simulink model "TMR_Model"  (R2024a)
settings: Solver=FixedStepAuto  StartTime=0.0  StopTime=10.0  RelTol=1e-3
settings OptimizationCC: DefaultParameterBehavior=Inlined  UseDivisionForNetSlopeComputation=on  GainParamInheritBuiltInType=on  UseFloatMulNetSlope=on  InlineInvariantSignals=on  PassReuseOutputArgsAs=Individual arguments  ZeroExternalMemoryAtStartup=off  ZeroInternalMemoryAtStartup=off  NoFixptDivByZeroProtection=on  EfficientFloat2IntCast=on  LifeSpan=1  OptimizeBlockOrder=speed  DifferentSizesBufferReuse=on  EfficientTunableParamExpr=on
settings DebuggingCC: ParameterTunabilityLossMsg=error
settings HardwareCC: ProdBitPerInt=16  ProdBitPerPointer=16  ProdBitPerSizeT=16  ProdBitPerPtrDiffT=16  ProdLargestAtomicFloat=None  ProdWordSize=8  ProdLongLongMode=on  ProdHWDeviceType=Atmel->AVR
settings SFSimCC: MATLABDynamicMemAlloc=off
settings RTWCC: Description=Embedded Coder  SystemTargetFile=ert.tlc  TemplateMakefile=ert_default_tmf
settings CodeAppCC: ForceParamTrailComments=on  IgnoreCustomStorageClasses=off  OperatorAnnotations=on  SimulinkDataObjDesc=on  SFDataObjDesc=on  CustomSymbolStrGlobalVar=rt$N$M  CustomSymbolStrType=$N$M  CustomSymbolStrFcn=$N$M$F  CustomSymbolStrMacro=$N$M  InsertBlockDesc=on
settings ERTTargetCC: TargetLangStandard=C99 (ISO)  GenerateSampleERTMain=on  IncludeMdlTerminateFcn=off  CombineSignalStateStructs=on  SupportAbsoluteTime=off  SupportComplex=off  SupportContinuousTime=on  InlinedParameterPlacement=NonHierarchical  ERTCustomFileTemplate=example_file_process.tlc  ERTFilePackagingFormat=CompactWithDataFile

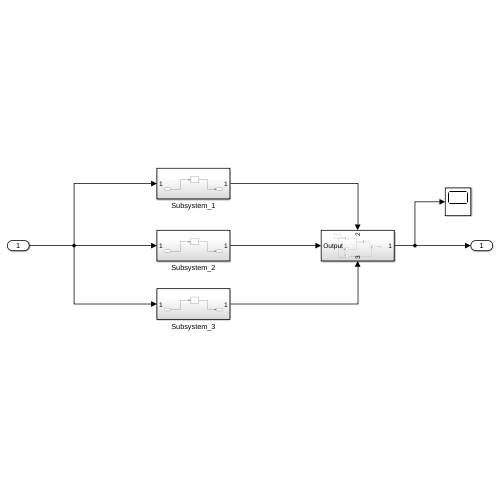
[thumbnail: Simulink's stored preview of the top-level diagram]
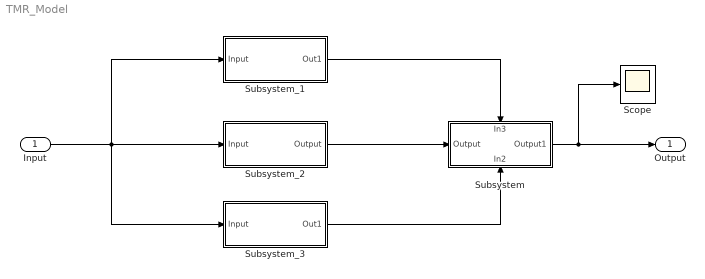
== system TMR_Model ==
  Input : Inport
  Scope : Scope
  Subsystem : Subsystem
      settings: PortSchema="{\"entries\":[{\"content\":{\"sides\":[{\"content\":{\"connectorIds\":[\"In1\"]},\"type\":\"ConnectorPlacement.EquallySpacedRectSide\",\"uuid\":\"1f9a2672-6573-4709-8234-f598f1a5eca2\"},{\"content\":{\"connectorIds\":[\"Out1\"],\"side\":\"RIGHT\"},\"type\":\"ConnectorPlacement.EquallySpacedRectSide\",\"uuid\":\"a731a0e8-5849-4b2b-a373-96344aad8381\"},{\"content\":{\"connectorIds\":[\"In2\"],\"side\":\"TOP\"},\"type\":\"ConnectorPlacement.EquallySpacedRectSide\",\"uuid\":\"49a1570a-9911-44de-ab8f-484fa4b3fc8c\"},{\"content\":{\"connectorIds\":[\"In3\"],\"side\":\"BOTTOM\"},\"type\":\"ConnectorPlacement.EquallySpacedRectSide\",\"uuid\":\"abd30324-337e-4863-944b-5764d9385d12\"}]},\"type\":\"ConnectorPlacement.EquallySpacedConnector\",\"uuid\":\"7aff7d2f-8702-452e-8e48-0fd052e56163\"}],\"packageUris\":[\"http://schema.mathworks.com/mf0/Connector/R2020b\"],\"version\":\"1.0\"}"
  Subsystem_1 : Subsystem
  Subsystem_2 : Subsystem
  Subsystem_3 : Subsystem
  Output : Outport
  wires:
  Input/1 -> Subsystem_3/1(Input), Subsystem_1/1(Input), Subsystem_2/1(Input)
  Subsystem_1/1(Out1) -> Subsystem/2(In3)
  Subsystem_2/1(Output) -> Subsystem/1(Output)
  Subsystem_3/1(Out1) -> Subsystem/3(In2)
  Subsystem/1(Output1) -> Scope/1, Output/1

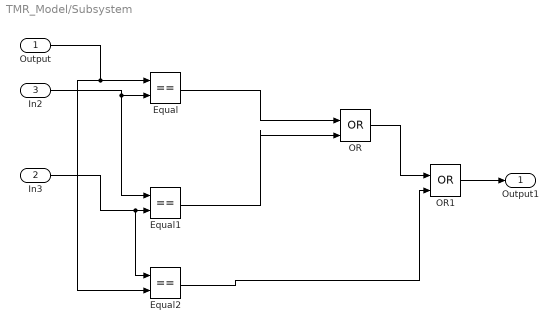
== system TMR_Model/Subsystem ==
  Output : Inport
  In3 : Inport  Port=2
  In2 : Inport  Port=3
  Equal : RelationalOperator  Operator===  OutDataTypeStr=boolean  RndMeth=Simplest  InputSameDT=off
  Equal1 : RelationalOperator  Operator===  OutDataTypeStr=boolean  RndMeth=Simplest  InputSameDT=off
  Equal2 : RelationalOperator  Operator===  OutDataTypeStr=boolean  RndMeth=Simplest  InputSameDT=off
  OR : Logic  Operator=OR  IconShape=distinctive  AllPortsSameDT=off  OutDataTypeStr=boolean
  OR1 : Logic  Operator=OR  IconShape=distinctive  AllPortsSameDT=off  OutDataTypeStr=boolean
  Output1 : Outport
  wires:
  Output/1 -> Equal/1, Equal2/2
  In2/1 -> Equal/2, Equal1/1
  In3/1 -> Equal2/1, Equal1/2
  Equal1/1 -> OR/2
  Equal/1 -> OR/1
  Equal2/1 -> OR1/2
  OR/1 -> OR1/1
  OR1/1 -> Output1/1

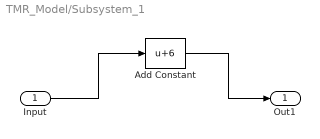
== system TMR_Model/Subsystem_1 ==
  Input : Inport
  Add Constant : Bias  Bias=6  SaturateOnIntegerOverflow=off
  Out1 : Outport
  wires:
  Input/1 -> Add Constant/1
  Add Constant/1 -> Out1/1

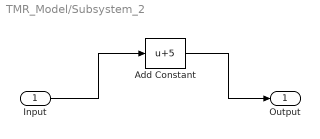
== system TMR_Model/Subsystem_2 ==
  Input : Inport
  Add Constant : Bias  Bias=5  SaturateOnIntegerOverflow=off
  Output : Outport
  wires:
  Input/1 -> Add Constant/1
  Add Constant/1 -> Output/1

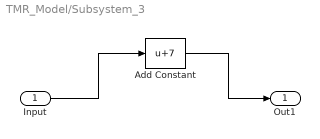
== system TMR_Model/Subsystem_3 ==
  Input : Inport
  Add Constant : Bias  Bias=7  SaturateOnIntegerOverflow=off
  Out1 : Outport
  wires:
  Input/1 -> Add Constant/1
  Add Constant/1 -> Out1/1
